simulink model "lungs_compliance"  (R2020b)
settings: Solver=VariableStepAuto  StartTime=0.0  StopTime=4  MaxStep=1e-3  RelTol=1e-3
model workspace (MAT data in the model file):
  E = 9.1
  Em = 60
  Kf = 0.8
  Kv = -0.6
  R0 = 0.1
  Rm = 0.85
  Vdot_max = 50
  Vdot_min = -70
settings Model: Creator=upattacini  LastModifiedBy=upattacini
settings DataIOCC: SaveFormat=StructureWithTime  SignalLogging=off  DSMLogging=off  SaveTime=off  ReturnWorkspaceOutputs=off

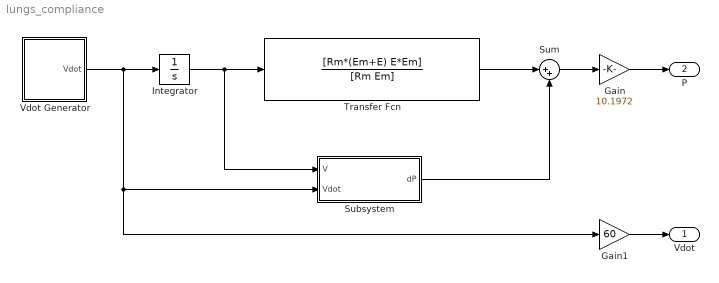
== system lungs_compliance ==
  Gain : Gain  Gain=10.1972
  Gain1 : Gain  Gain=60
  Integrator : Integrator
  Subsystem : Subsystem
  Sum : Sum  Inputs=|++
  Transfer Fcn : TransferFcn  Numerator=[Rm*(Em+E) E*Em]  Denominator=[Rm Em]
  Vdot Generator : Subsystem
  Vdot : Outport
  P : Outport  Port=2
  wires:
  Vdot Generator/1(Vdot) -> Gain1/1, Subsystem/2(Vdot), Integrator/1
  Integrator/1 -> Subsystem/1(V), Transfer Fcn/1
  Transfer Fcn/1 -> Sum/1
  Subsystem/1(dP) -> Sum/2
  Sum/1 -> Gain/1
  Gain/1 -> P/1
  Gain1/1 -> Vdot/1

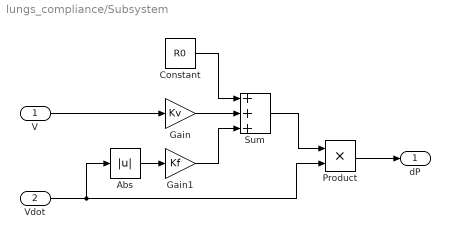
== system lungs_compliance/Subsystem ==
  V : Inport
  Vdot : Inport  Port=2
  Abs : Abs
  Constant : Constant  Value=R0
  Gain : Gain  Gain=Kv
  Gain1 : Gain  Gain=Kf
  Product : Product
  Sum : Sum  Inputs=3
  dP : Outport
  wires:
  Product/1 -> dP/1
  Vdot/1 -> Product/2, Abs/1
  Constant/1 -> Sum/1
  V/1 -> Gain/1
  Gain/1 -> Sum/2
  Gain1/1 -> Sum/3
  Sum/1 -> Product/1
  Abs/1 -> Gain1/1

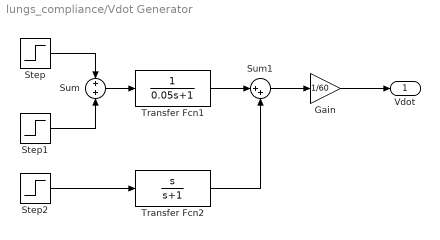
== system lungs_compliance/Vdot Generator ==
  Gain : Gain  Gain=1/60
  Step : Step  Time=0.5  After=Vdot_max  SampleTime=0
  Step1 : Step  Time=1.5  After=-Vdot_max  SampleTime=0
  Step2 : Step  Time=2.2  After=Vdot_min  SampleTime=0
  Sum : Sum
  Sum1 : Sum  Inputs=|++
  Transfer Fcn1 : TransferFcn  Denominator=[0.05 1]
  Transfer Fcn2 : TransferFcn  Numerator=[1 0]  Denominator=[1 1]
  Vdot : Outport
  wires:
  Sum/1 -> Transfer Fcn1/1
  Step/1 -> Sum/1
  Step1/1 -> Sum/2
  Transfer Fcn1/1 -> Sum1/1
  Sum1/1 -> Gain/1
  Transfer Fcn2/1 -> Sum1/2
  Step2/1 -> Transfer Fcn2/1
  Gain/1 -> Vdot/1
